simulink model "Calculator_Harness"  (R2020b)
settings: configuration reference "FixedStepConfig" (kept outside this file)
settings Model: Creator=sk71149  LastModifiedBy=sk71149
settings ConfigSetRef: SourceName=FixedStepConfig  SourceLocation=Base Workspace

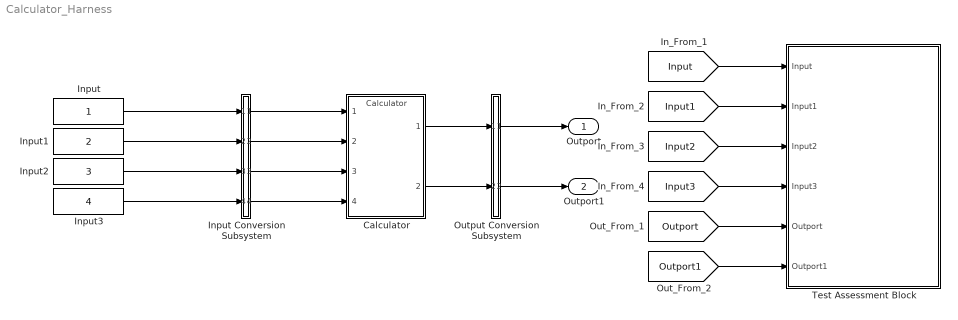
== system Calculator_Harness ==
  Calculator : ModelReference  ModelNameDialog=Calculator  SimulationMode=Normal  ModelReferenceVersion=1.5
  Input : Constant  OutDataTypeStr=double  SampleTime=0.01
  Input Conversion Subsystem : Subsystem  Tag=__SLT_ICS__  Description=|
      | Signal spec.
      | and routing
      settings: AttributesFormatString=%<Description>
  Input1 : Constant  Value=2  OutDataTypeStr=double  SampleTime=0.01
  Input2 : Constant  Value=3  OutDataTypeStr=double  SampleTime=0.01
  Input3 : Constant  Value=4  OutDataTypeStr=double  SampleTime=0.01
  Output Conversion Subsystem : Subsystem  Tag=__SLT_OCS__  Description=|
      | Signal spec.
      | and routing
      settings: AttributesFormatString=%<Description>
  Test Assessment Block : Test Sequence  Tag=__SLT_ASMT__  TreatAsAtomicUnit=on
  Outport : Outport
  Outport1 : Outport  Port=2
  wires:
  [Input] -> Test Assessment Block/1(Input)
  [Input1] -> Test Assessment Block/2(Input1)
  [Input2] -> Test Assessment Block/3(Input2)
  [Input3] -> Test Assessment Block/4(Input3)
  [Outport] -> Test Assessment Block/5(Outport)
  [Outport1] -> Test Assessment Block/6(Outport1)
  Input/1 -> Input Conversion Subsystem/1(Inport_1)
  Input1/1 -> Input Conversion Subsystem/2(Inport_2)
  Input2/1 -> Input Conversion Subsystem/3(Inport_3)
  Input3/1 -> Input Conversion Subsystem/4(Inport_4)
  Output Conversion Subsystem/1(Outport_1) -> Outport/1
  Output Conversion Subsystem/2(Outport_2) -> Outport1/1
  Input Conversion Subsystem/1(Outport_1) -> Calculator/1
  Input Conversion Subsystem/2(Outport_2) -> Calculator/2
  Input Conversion Subsystem/3(Outport_3) -> Calculator/3
  Input Conversion Subsystem/4(Outport_4) -> Calculator/4
  Calculator/1 -> Output Conversion Subsystem/1(Inport_1)
  Calculator/2 -> Output Conversion Subsystem/2(Inport_2)

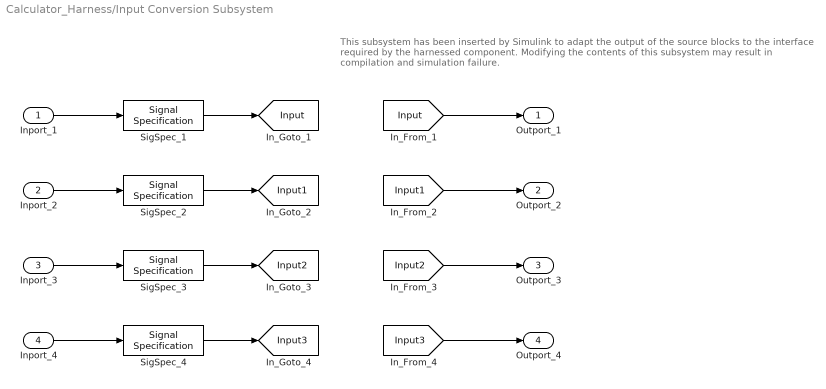
== system Calculator_Harness/Input Conversion Subsystem ==
  note: This subsystem has been inserted by Simulink to adapt the output of the source blocks to the interface required by the harnessed component.
      |  Modifying the contents of this subsystem may result in compilation and simulation failure.
  Inport_1 : Inport
  Inport_2 : Inport  Port=2
  Inport_3 : Inport  Port=3
  Inport_4 : Inport  Port=4
  SigSpec_{1..4} (4 alike) : SignalSpecification  OutDataTypeStr=double  Dimensions=[1]  SampleTime=0.01
  Outport_1 : Outport
  Outport_2 : Outport  Port=2
  Outport_3 : Outport  Port=3
  Outport_4 : Outport  Port=4
  tag scope: Input1=global, Input2=global, Input3=global, Input=global
  wires:
  [Input] -> Outport_1/1
  SigSpec_1/1 -> [Input]
  Inport_1/1 -> SigSpec_1/1
  [Input1] -> Outport_2/1
  SigSpec_2/1 -> [Input1]
  Inport_2/1 -> SigSpec_2/1
  [Input2] -> Outport_3/1
  SigSpec_3/1 -> [Input2]
  Inport_3/1 -> SigSpec_3/1
  [Input3] -> Outport_4/1
  SigSpec_4/1 -> [Input3]
  Inport_4/1 -> SigSpec_4/1

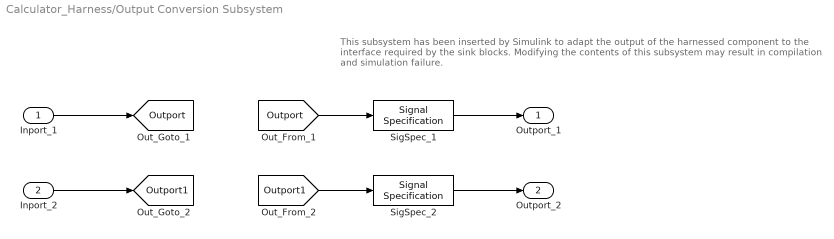
== system Calculator_Harness/Output Conversion Subsystem ==
  note: This subsystem has been inserted by Simulink to adapt the output of the harnessed component to the interface required by the sink blocks.
      |  Modifying the contents of this subsystem may result in compilation and simulation failure.
  Inport_1 : Inport
  Inport_2 : Inport  Port=2
  SigSpec_1 : SignalSpecification  OutDataTypeStr=double  Dimensions=[1]  SampleTime=0.01
  SigSpec_2 : SignalSpecification  OutDataTypeStr=double  Dimensions=[1]  SampleTime=0.01
  Outport_1 : Outport
  Outport_2 : Outport  Port=2
  tag scope: Outport1=global, Outport=global
  wires:
  Inport_1/1 -> [Outport]
  [Outport] -> SigSpec_1/1
  SigSpec_1/1 -> Outport_1/1
  Inport_2/1 -> [Outport1]
  [Outport1] -> SigSpec_2/1
  SigSpec_2/1 -> Outport_2/1

== stateflow chart Calculator_Harness/Test Assessment Block ==
  settings: stateMachineType=SIMPLIFIED_MACHINE
  state verify_statements
    verify(Outport1==3)
    verify(Outport == 12)
  (default) -> verify_statements
  data: Input input double size=[1]; Input1 input double size=[1]; Input2 input double size=[1]; Input3 input double size=[1]; Outport input double size=[1]; Outport1 input double size=[1]
